simulink model "rate_saturator_mdl"  (Simulink 5.1)
settings: Solver=ode4  SolverMode=SingleTasking  StartTime=0.0  StopTime=tdur  FixedStep=dt  RelTol=1e-3
values from neighbouring files (symbols this model uses):
  dt = 0.1    [attitude_controller_response.m]
  I = I_array(ax)    [attitude_controller_response.m]
  Kd = Kd_array(ax)    [attitude_controller_response.m]
  Krcs = 1    [attitude_controller_response.m]
  Tdist = Tdist_array(ax)    [attitude_controller_response.m]
  Trcs_max = Trcs_max_array(ax)    [attitude_controller_response.m]
libraries: simulink_extras x1
settings Model: LastModifiedBy=Sean Hardacre  SaveOutput=off  LimitDataPoints=off  BooleanDataType=on  ProdHWDeviceType=Microprocessor

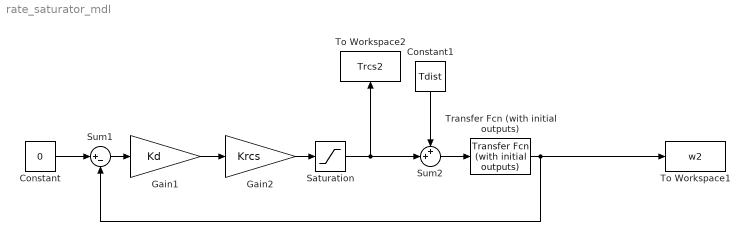
== system rate_saturator_mdl ==
  Constant : Constant  Value=0
  Constant1 : Constant  Orientation=down  Value=Tdist
  Gain1 : Gain  Gain=Kd  SaturateOnIntegerOverflow=on
  Gain2 : Gain  Gain=Krcs  SaturateOnIntegerOverflow=on
  Saturation : Saturate  UpperLimit=Trcs_max  LowerLimit=-Trcs_max  SampleTime=dt
  Sum1 : Sum  Inputs=|+-  SaturateOnIntegerOverflow=on
  Sum2 : Sum  Inputs=++|  SaturateOnIntegerOverflow=on
  To Workspace1 : ToWorkspace  VariableName=w2  SampleTime=dt  SaveFormat=Array
  To Workspace2 : ToWorkspace  VariableName=Trcs2  SampleTime=dt  SaveFormat=Array
      settings: Orientation=up
  Transfer Fcn (with initial outputs) : simulink_extras/Additional Linear/Transfer Fcn (with initial outputs)  N=[1]  D=[I 0]  Y0=w0  U0=0
  wires:
  Constant/1 -> Sum1/1
  Sum1/1 -> Gain1/1
  Gain1/1 -> Gain2/1
  Transfer Fcn (with initial outputs)/1 -> Sum1/2, To Workspace1/1
  Sum2/1 -> Transfer Fcn (with initial outputs)/1
  Gain2/1 -> Saturation/1
  Constant1/1 -> Sum2/1
  Saturation/1 -> Sum2/2, To Workspace2/1
